simulink model "sf_fixpt"  (Simulink 6.0)
settings: Solver=ode45  StartTime=0.0  StopTime=1  RelTol=1e-3
settings Model: CovMetricSettings=dcmtr  Creator=The MathWorks Inc.  LastModifiedBy=batserve  ExtModeAutoUpdateStatusClock=off
settings DataIOCC: SignalLoggingName=sigsOut
settings DebuggingCC: CheckExecutionContextPreStartOutputMsg=on  CheckExecutionContextRuntimeOutputMsg=on  SolverPrmCheckMsg=none
settings HardwareCC: TargetUnknown=on

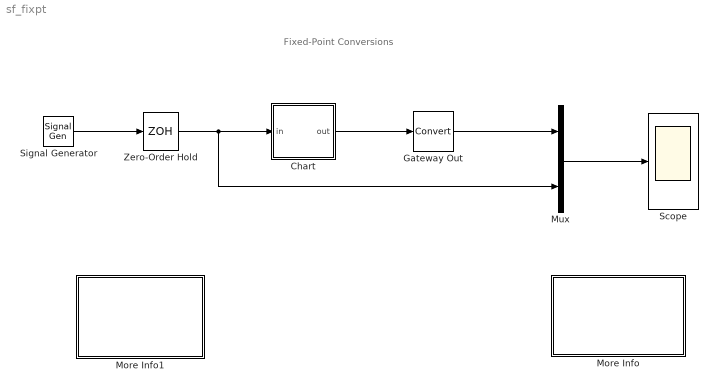
== system sf_fixpt ==
  note: Fixed-Point Conversions
  Chart : Stateflow chart  PropExecContextAcrossSSBoundary=on
  Gateway Out : DataTypeConversion  OutDataTypeMode=double
  More Info : Subsystem  PropExecContextAcrossSSBoundary=on
      mask Display: disp('Double click\nhere for\ninformation on\nthis demonstration')
  More Info1 : Subsystem  PropExecContextAcrossSSBoundary=on
      settings: OpenFcn=simcad(bdroot);
      mask Display: disp('Double click\nhere for\nSimulink\Stateflow\n Help')
  Mux : Mux  Inputs=2
  Scope : Scope
      settings: TimeRange=1  YMin=-10  YMax=10
  Signal Generator : SignalGenerator  WaveForm=sawtooth  Amplitude=10
  Zero-Order Hold : ZeroOrderHold  SampleTime=.001
  wires:
  Chart/1(out) -> Gateway Out/1
  Signal Generator/1 -> Zero-Order Hold/1
  Zero-Order Hold/1 -> Chart/1(in), Mux/2
  Gateway Out/1 -> Mux/1
  Mux/1 -> Scope/1

== system sf_fixpt/More Info ==
  note: Fixed-Point Multiplication
  note: Stateflow allows you to include fixed-point data in your chart. This demonstration illustrates
      | how you can input a value of type 'double' to a stateflow chart and output a fixed-point data
      | type back to Simulink. The output data type is an 8 bit signed integer with a  slope bias of 2^-5.
      | This means that the maximum value of the output is 3.96875 and the minimum value is -4.
      |
      | If you run the simulation, you will notice that chart output signal truncates the input signal at the
      | above mentioned maximum and minimum values. The Stateflow chart is simply taking the input
      | signal and changing the data type to fixed point. This allows you to use the Stateflow chart as
      | a fixed-point data converter.

== system sf_fixpt/More Info1 ==

== stateflow chart Chart ==
  note: Note: Converting a double to a fixpt type
      | contains an inherent overflow and this
      | is detected by the Stateflow Debugger.
      | For illustrative purposes, this data-range
      | check is turned off in the Stateflow Debugger.
  (default) -> (junction 4) : {out=in;}
  data: in input double; out output fixpt
